simulink library "relay_ANSI_functions_lib"  (Simulink 8.1)
settings: Solver=ode45  StartTime=0.0  StopTime=10.0  RelTol=1e-3
values from neighbouring files (symbols this model uses):
  Ts = 100E-6    (= 0.0001)    [UnitTest_relay_model_init.m]    (also in relay_settings_init.m)
undefined symbols (not defined in the file or in its folder): IOC, TOC, VRMSLL
libraries: simulink x4
settings Model: Creator=RE25624  LastModifiedBy=re25624

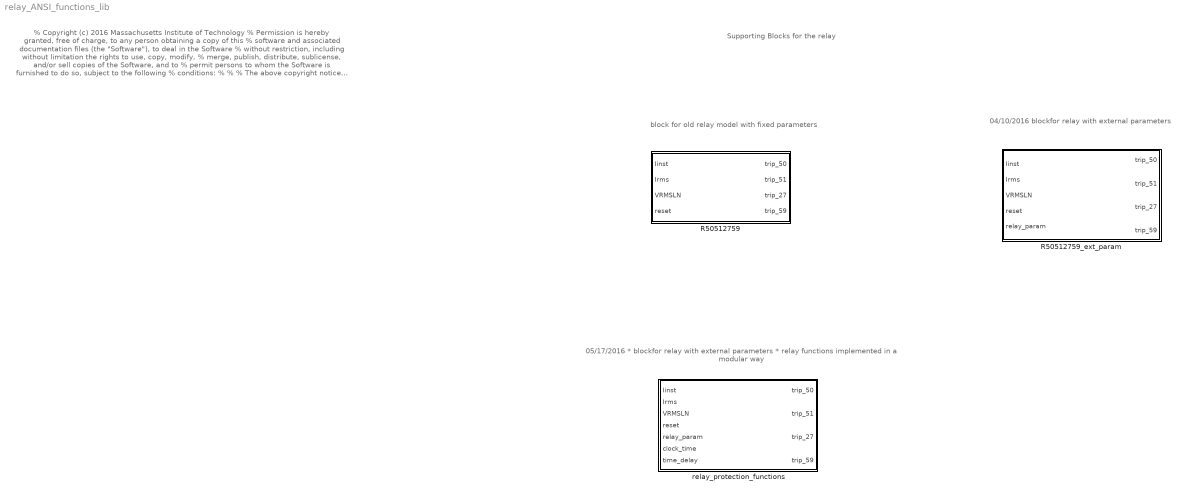
== system relay_ANSI_functions_lib ==
  note: 04/10/2016
      | blockfor relay with external parameters
  note: Supporting Blocks for the relay
  note: block for old relay model with fixed parameters
  note: 05/17/2016
      | * blockfor relay with external parameters
      | * relay functions implemented in a modular way
  note: % Copyright (c) 2016 Massachusetts Institute of Technology
      | % Permission is hereby granted, free of charge, to any person obtaining a copy of this
      | % software and associated documentation files (the "Software"), to deal in the Software
      | % without restriction, including without limitation the rights to use, copy, modify,
      | % merge, publish, distribute, sublicense, and/or sell copies of the Software, and to
      | % permit persons to whom the Software is furnished to do so, subject to the following
      | % conditions:
      | %
      | %
      | % The above copyright notice and this permission notice shall be included in
      | % all copies or substantial portions of the Software.
      | %
      | % THE SOFTWARE IS PROVIDED "AS IS", WITHOUT WARRANTY OF ANY KIND, EXPRESS OR IMPLIED,
      | % INCLUDING BUT NOT LIMITED TO THE WARRANTIES OF MERCHANTABILITY, FITNESS FOR A
      | % PARTICULAR PURPOSE AND NONINFRINGEMENT. IN NO EVENT SHALL THE AUTHORS OR COPYRIGHT
      | % HOLDERS BE LIABLE FOR ANY CLAIM, DAMAGES OR OTHER LIABILITY, WHETHER IN AN ACTION
      | % OF CONTRACT, TORT OR OTHERWISE, ARISING FROM, OUT OF OR IN CONNECTION WITH THE
      | % SOFTWARE OR THE USE OR OTHER DEALINGS IN THE SOFTWARE.
      | %
      | %
      | %%
  R50512759 : Subsystem  mask(Relays 50-51-27-59){VRMSLL=VRMSLL, IOC=IOC, TOC=TOC, Ts=Ts}
      mask prompts: VRMSLL "Nominal Voltage [VRMSLL]"; IOC "IOC Setting [A]"; TOC "TOC Setting [A]"; Ts "Sampling Time [Sec]"
      mask help:
      | This block simulates the behavior of the following relay functions:
      | 1) Instantaneous overcurrent (50)
      | 2) AC inverse time overcurrent (51)
      | 3) Undervoltage (27)
      | 4) Overvoltage (59)
      | It is not suitable for instantaneous earth current relaying.
      | The model neglects the influence CTs since only the logics of the relay are required or the current effort.
  R50512759_ext_param : Subsystem  mask(Relays 50-51-27-59){Ts=Ts}
      mask prompts: Ts "Sampling Time [Sec]"
      mask help:
      | This block simulates the behavior of the following relay functions:
      | 1) Instantaneous overcurrent (50)
      | 2) AC inverse time overcurrent (51)
      | 3) Undervoltage (27)
      | 4) Overvoltage (59)
      | It is not suitable for instantaneous earth current relaying.
      | The model neglects the influence CTs since only the logics of the relay are required or the current effort.
      |
      | The input bus with the relay parameters should be ordered as follows:
      | 1) VRMSLL
      | 2) IOC
      | 3) TOC
      | 4) dV_threshold
      | 5) angle_threshold
      | 6) dF_threshold
  relay_protection_functions : Subsystem  mask(Relays 50-51-27-59){Ts=Ts}
      mask prompts: Ts "Sampling Time [Sec]"
      mask help:
      | This block simulates the behavior of the following relay functions:
      | 1) Instantaneous overcurrent (50)
      | 2) AC inverse time overcurrent (51)
      | 3) Undervoltage (27)
      | 4) Overvoltage (59)
      | It is not suitable for instantaneous earth current relaying.
      | The model neglects the influence CTs since only the logics of the relay are required or the current effort.
      |
      | The input bus with the relay parameters should be ordered as follows:
      | 1) VRMSLL
      | 2) IOC
      | 3) TOC
      | 4) dV_threshold
      | 5) angle_threshold
      | 6) dF_threshold

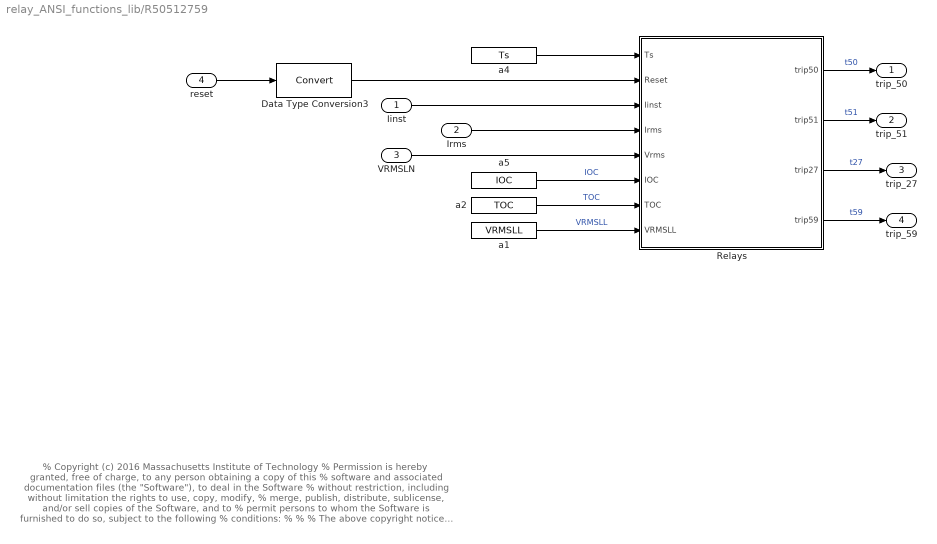
== system relay_ANSI_functions_lib/R50512759 ==
  note: % Copyright (c) 2016 Massachusetts Institute of Technology
      | % Permission is hereby granted, free of charge, to any person obtaining a copy of this
      | % software and associated documentation files (the "Software"), to deal in the Software
      | % without restriction, including without limitation the rights to use, copy, modify,
      | % merge, publish, distribute, sublicense, and/or sell copies of the Software, and to
      | % permit persons to whom the Software is furnished to do so, subject to the following
      | % conditions:
      | %
      | %
      | % The above copyright notice and this permission notice shall be included in
      | % all copies or substantial portions of the Software.
      | %
      | % THE SOFTWARE IS PROVIDED "AS IS", WITHOUT WARRANTY OF ANY KIND, EXPRESS OR IMPLIED,
      | % INCLUDING BUT NOT LIMITED TO THE WARRANTIES OF MERCHANTABILITY, FITNESS FOR A
      | % PARTICULAR PURPOSE AND NONINFRINGEMENT. IN NO EVENT SHALL THE AUTHORS OR COPYRIGHT
      | % HOLDERS BE LIABLE FOR ANY CLAIM, DAMAGES OR OTHER LIABILITY, WHETHER IN AN ACTION
      | % OF CONTRACT, TORT OR OTHERWISE, ARISING FROM, OUT OF OR IN CONNECTION WITH THE
      | % SOFTWARE OR THE USE OR OTHER DEALINGS IN THE SOFTWARE.
      | %
      | %
      | %%
  Iinst : Inport
  Irms : Inport  Port=2
  VRMSLN : Inport  Port=3
  reset : Inport  Port=4
  Data Type Conversion3 : DataTypeConversion
  Relays : MATLAB Function  TreatAsAtomicUnit=on
  a1 : Constant  Value=VRMSLL
  a2 : Constant  Value=TOC
  a4 : Constant  Value=Ts
  a5 : Constant  Value=IOC
  trip_50 : Outport
  trip_51 : Outport  Port=2
  trip_27 : Outport  Port=3
  trip_59 : Outport  Port=4
  wires:
  Data Type Conversion3/1 -> Relays/2(Reset)
  Relays/2(trip51) -> trip_51/1  "t51"
  Relays/1(trip50) -> trip_50/1  "t50"
  Relays/4(trip59) -> trip_59/1  "t59"
  Relays/3(trip27) -> trip_27/1  "t27"
  a4/1 -> Relays/1(Ts)
  a1/1 -> Relays/8(VRMSLL)  "VRMSLL"
  VRMSLN/1 -> Relays/5(Vrms)
  Irms/1 -> Relays/4(Irms)
  a2/1 -> Relays/7(TOC)  "TOC"
  Iinst/1 -> Relays/3(Iinst)
  a5/1 -> Relays/6(IOC)  "IOC"
  reset/1 -> Data Type Conversion3/1

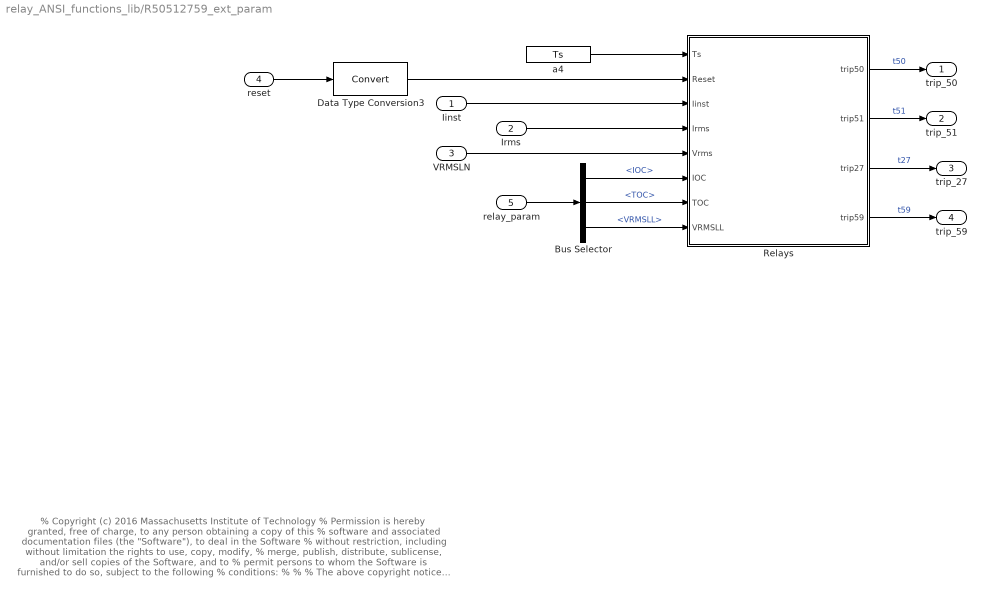
== system relay_ANSI_functions_lib/R50512759_ext_param ==
  note: % Copyright (c) 2016 Massachusetts Institute of Technology
      | % Permission is hereby granted, free of charge, to any person obtaining a copy of this
      | % software and associated documentation files (the "Software"), to deal in the Software
      | % without restriction, including without limitation the rights to use, copy, modify,
      | % merge, publish, distribute, sublicense, and/or sell copies of the Software, and to
      | % permit persons to whom the Software is furnished to do so, subject to the following
      | % conditions:
      | %
      | %
      | % The above copyright notice and this permission notice shall be included in
      | % all copies or substantial portions of the Software.
      | %
      | % THE SOFTWARE IS PROVIDED "AS IS", WITHOUT WARRANTY OF ANY KIND, EXPRESS OR IMPLIED,
      | % INCLUDING BUT NOT LIMITED TO THE WARRANTIES OF MERCHANTABILITY, FITNESS FOR A
      | % PARTICULAR PURPOSE AND NONINFRINGEMENT. IN NO EVENT SHALL THE AUTHORS OR COPYRIGHT
      | % HOLDERS BE LIABLE FOR ANY CLAIM, DAMAGES OR OTHER LIABILITY, WHETHER IN AN ACTION
      | % OF CONTRACT, TORT OR OTHERWISE, ARISING FROM, OUT OF OR IN CONNECTION WITH THE
      | % SOFTWARE OR THE USE OR OTHER DEALINGS IN THE SOFTWARE.
      | %
      | %
      | %%
  Iinst : Inport
  Irms : Inport  Port=2
  VRMSLN : Inport  Port=3
  reset : Inport  Port=4
  relay_param : Inport  Port=5
  Bus Selector : BusSelector  OutputSignals=IOC,TOC,VRMSLL
  Data Type Conversion3 : DataTypeConversion
  Relays : MATLAB Function  TreatAsAtomicUnit=on
  a4 : Constant  Value=Ts
  trip_50 : Outport
  trip_51 : Outport  Port=2
  trip_27 : Outport  Port=3
  trip_59 : Outport  Port=4
  wires:
  relay_param/1 -> Bus Selector/1
  Data Type Conversion3/1 -> Relays/2(Reset)
  Relays/2(trip51) -> trip_51/1  "t51"
  Relays/1(trip50) -> trip_50/1  "t50"
  Relays/4(trip59) -> trip_59/1  "t59"
  Relays/3(trip27) -> trip_27/1  "t27"
  a4/1 -> Relays/1(Ts)
  Bus Selector/3 -> Relays/8(VRMSLL)  "<VRMSLL>"
  VRMSLN/1 -> Relays/5(Vrms)
  Irms/1 -> Relays/4(Irms)
  Bus Selector/2 -> Relays/7(TOC)  "<TOC>"
  Iinst/1 -> Relays/3(Iinst)
  Bus Selector/1 -> Relays/6(IOC)  "<IOC>"
  reset/1 -> Data Type Conversion3/1

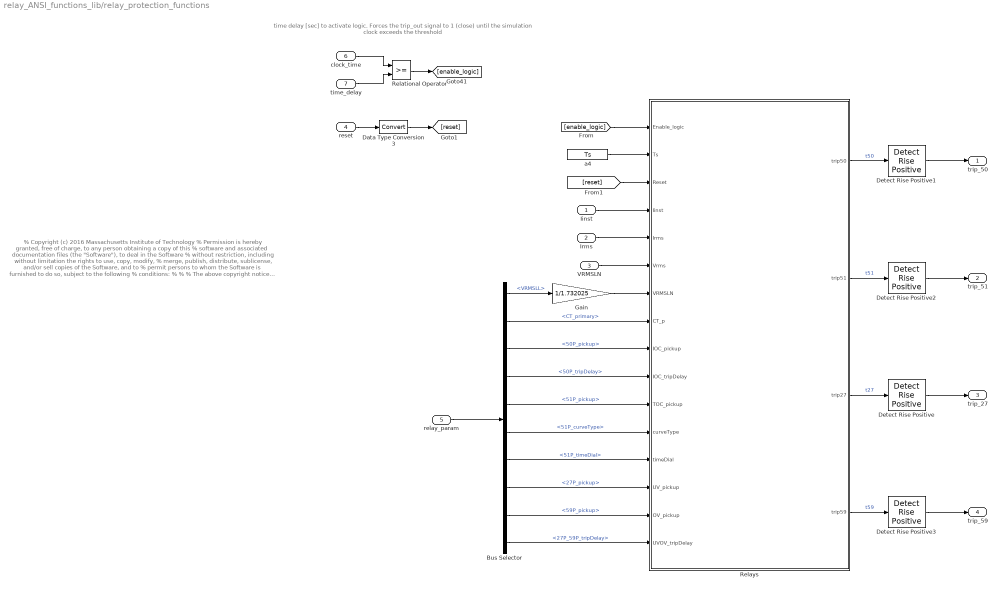
== system relay_ANSI_functions_lib/relay_protection_functions ==
  note: time delay [sec] to activate logic. Forces the trip_out signal
      | to 1 (close) until the simulation clock exceeds the threshold
  note: % Copyright (c) 2016 Massachusetts Institute of Technology
      | % Permission is hereby granted, free of charge, to any person obtaining a copy of this
      | % software and associated documentation files (the "Software"), to deal in the Software
      | % without restriction, including without limitation the rights to use, copy, modify,
      | % merge, publish, distribute, sublicense, and/or sell copies of the Software, and to
      | % permit persons to whom the Software is furnished to do so, subject to the following
      | % conditions:
      | %
      | %
      | % The above copyright notice and this permission notice shall be included in
      | % all copies or substantial portions of the Software.
      | %
      | % THE SOFTWARE IS PROVIDED "AS IS", WITHOUT WARRANTY OF ANY KIND, EXPRESS OR IMPLIED,
      | % INCLUDING BUT NOT LIMITED TO THE WARRANTIES OF MERCHANTABILITY, FITNESS FOR A
      | % PARTICULAR PURPOSE AND NONINFRINGEMENT. IN NO EVENT SHALL THE AUTHORS OR COPYRIGHT
      | % HOLDERS BE LIABLE FOR ANY CLAIM, DAMAGES OR OTHER LIABILITY, WHETHER IN AN ACTION
      | % OF CONTRACT, TORT OR OTHERWISE, ARISING FROM, OUT OF OR IN CONNECTION WITH THE
      | % SOFTWARE OR THE USE OR OTHER DEALINGS IN THE SOFTWARE.
      | %
      | %
      | %%
  Iinst : Inport
  Irms : Inport  Port=2
  VRMSLN : Inport  Port=3
  reset : Inport  Port=4
  relay_param : Inport  Port=5
  clock_time : Inport  Port=6
  time_delay : Inport  Port=7
  Bus Selector : BusSelector  OutputSignals=VRMSLL,CT_primary,50P_pickup,50P_tripDelay,51P_pickup,51P_curveType,51P_timeDial,27P_pickup,59P_pickup,27P_59P_tripDelay
  Data Type Conversion3 : DataTypeConversion
  Detect Rise Positive{,1..3} (4 alike) : simulink/Logic and Bit Operations/Detect Rise Positive  vinit=0  InputProcessing=Inherited  OutDataTypeStr=boolean
  Gain : Gain  Gain=1/1.732025
  Relational Operator : RelationalOperator  OutDataTypeStr=boolean
  Relays : MATLAB Function  TreatAsAtomicUnit=on
  a4 : Constant  Value=Ts
  trip_50 : Outport
  trip_51 : Outport  Port=2
  trip_27 : Outport  Port=3
  trip_59 : Outport  Port=4
  wires:
  Detect Rise Positive3/1 -> trip_59/1
  Detect Rise Positive/1 -> trip_27/1
  Detect Rise Positive2/1 -> trip_51/1
  Detect Rise Positive1/1 -> trip_50/1
  Relays/4(trip59) -> Detect Rise Positive3/1  "t59"
  Relays/2(trip51) -> Detect Rise Positive2/1  "t51"
  Relays/1(trip50) -> Detect Rise Positive1/1  "t50"
  Relays/3(trip27) -> Detect Rise Positive/1  "t27"
  [reset] -> Relays/3(Reset)
  Data Type Conversion3/1 -> [reset]
  Gain/1 -> Relays/7(VRMSLN)
  Bus Selector/8 -> Relays/14(UV_pickup)  "<27P_pickup>"
  Bus Selector/9 -> Relays/15(OV_pickup)  "<59P_pickup>"
  Bus Selector/10 -> Relays/16(UVOV_tripDelay)  "<27P_59P_tripDelay>"
  Iinst/1 -> Relays/4(Iinst)
  Irms/1 -> Relays/5(Irms)
  Bus Selector/7 -> Relays/13(timeDial)  "<51P_timeDial>"
  Bus Selector/6 -> Relays/12(curveType)  "<51P_curveType>"
  Bus Selector/5 -> Relays/11(TOC_pickup)  "<51P_pickup>"
  Bus Selector/4 -> Relays/10(IOC_tripDelay)  "<50P_tripDelay>"
  Bus Selector/3 -> Relays/9(IOC_pickup)  "<50P_pickup>"
  Bus Selector/2 -> Relays/8(CT_p)  "<CT_primary>"
  Bus Selector/1 -> Gain/1  "<VRMSLL>"
  reset/1 -> Data Type Conversion3/1
  VRMSLN/1 -> Relays/6(Vrms)
  a4/1 -> Relays/2(Ts)
  relay_param/1 -> Bus Selector/1
  clock_time/1 -> Relational Operator/1
  time_delay/1 -> Relational Operator/2
  Relational Operator/1 -> [enable_logic]
  [enable_logic] -> Relays/1(Enable_logic)

== matlab function relay_protection_functions/Relays ==
  data: Enable_logic input double; Ts input double; Reset input double; Iinst input double; Irms input double; Vrms input double; VRMSLN input double; CT_p input double; IOC_pickup input double; IOC_tripDelay input double; TOC_pickup input double; curveType input double; timeDial input double; UV_pickup input double; OV_pickup input double; UVOV_tripDelay input double; trip50 output double; trip51 output double; trip27 output double; trip59 output double
% Copyright (c) 2016 Massachusetts Institute of Technology
% Permission is hereby granted, free of charge, to any person obtaining a copy of this
% software and associated documentation files (the "Software"), to deal in the Software
% without restriction, including without limitation the rights to use, copy, modify,
% merge, publish, distribute, sublicense, and/or sell copies of the Software, and to
% permit persons to whom the Software is furnished to do so, subject to the following
% conditions:
%
%
% The above copyright notice and this permission notice shall be included in
% all copies or substantial portions of the Software.
%
% THE SOFTWARE IS PROVIDED "AS IS", WITHOUT WARRANTY OF ANY KIND, EXPRESS OR IMPLIED,
% INCLUDING BUT NOT LIMITED TO THE WARRANTIES OF MERCHANTABILITY, FITNESS FOR A
% PARTICULAR PURPOSE AND NONINFRINGEMENT. IN NO EVENT SHALL THE AUTHORS OR COPYRIGHT
% HOLDERS BE LIABLE FOR ANY CLAIM, DAMAGES OR OTHER LIABILITY, WHETHER IN AN ACTION
% OF CONTRACT, TORT OR OTHERWISE, ARISING FROM, OUT OF OR IN CONNECTION WITH THE
% SOFTWARE OR THE USE OR OTHER DEALINGS IN THE SOFTWARE.
%
%
%%

function [trip50, trip51, trip27, trip59] = relay_elements(Enable_logic, Ts, Reset, Iinst, Irms, Vrms, VRMSLN,...
    CT_p, IOC_pickup, IOC_tripDelay, TOC_pickup, curveType, timeDial, UV_pickup, OV_pickup, UVOV_tripDelay)
%#codegen

% initialize or reset the trip signals
persistent R50 R51 R27 R59
if isempty(R51) || Reset
    R50=false;
    R51=false;
    R59=false;
    R27=false;
end

% applying turns CT ratio - assuming protection type CT
Iinst = Iinst * (5/CT_p);
Irms = Irms * (5/CT_p);

% old- latch for true signals
% old- if ~(R50==true || R51==true) && Enable_logic==1
if Enable_logic==1
    % calling external function expressing relay protection elements
    T50 = relay_ANSI_50P_script(Ts, Iinst , IOC_pickup, IOC_tripDelay);
    T51 = relay_ANSI_51P_script(Ts, Irms, TOC_pickup, curveType, timeDial);
    T27 = relay_ANSI_27P_script(Ts, Vrms, VRMSLN, UV_pickup, UVOV_tripDelay);
    T59 = relay_ANSI_59P_script(Ts, Vrms, VRMSLN, OV_pickup, UVOV_tripDelay);
    
    R50 = T50;
    R51 = T51;
    R27 = T27;
    R59 = T59;
end

% external latch
trip50 = R50; % old- latched
trip51 = R51; % old- latched
trip27 = R27; % old- not latched
trip59 = R59; % old- not latched

== matlab function R50512759/Relays ==
  data: Ts input double; trip50 output double; Reset input double; Iinst input double; Irms input double; Vrms input double; IOC input double; trip51 output double; trip27 output double; TOC input double; VRMSLL input double; trip59 output double
% Copyright (c) 2016 Massachusetts Institute of Technology
% Permission is hereby granted, free of charge, to any person obtaining a copy of this 
% software and associated documentation files (the "Software"), to deal in the Software
% without restriction, including without limitation the rights to use, copy, modify, 
% merge, publish, distribute, sublicense, and/or sell copies of the Software, and to 
% permit persons to whom the Software is furnished to do so, subject to the following 
% conditions:
% 
% 
% The above copyright notice and this permission notice shall be included in 
% all copies or substantial portions of the Software.
% 
% THE SOFTWARE IS PROVIDED "AS IS", WITHOUT WARRANTY OF ANY KIND, EXPRESS OR IMPLIED, 
% INCLUDING BUT NOT LIMITED TO THE WARRANTIES OF MERCHANTABILITY, FITNESS FOR A 
% PARTICULAR PURPOSE AND NONINFRINGEMENT. IN NO EVENT SHALL THE AUTHORS OR COPYRIGHT 
% HOLDERS BE LIABLE FOR ANY CLAIM, DAMAGES OR OTHER LIABILITY, WHETHER IN AN ACTION 
% OF CONTRACT, TORT OR OTHERWISE, ARISING FROM, OUT OF OR IN CONNECTION WITH THE 
% SOFTWARE OR THE USE OR OTHER DEALINGS IN THE SOFTWARE.
%
%
%%


function [trip50, trip51, trip27, trip59] = relays_50512759(Ts, Reset, Iinst, Irms, Vrms, IOC, TOC, VRMSLL)
%#codegen

% initialize or reset the trip signals
persistent R50 R51 R27 R59
if isempty(R51) || Reset
    R50=false;
    R51=false;
    R59=false;
    R27=false;
end

% latch for true signals
if ~(R50==true || R51==true)
    % calling external function
    r = relay_ANSI_50512759_script(Ts, Iinst, Irms, Vrms, IOC, TOC, VRMSLL);
    R50 = r.trip50;
    R51 = r.trip51;
    R27 = r.trip27;
    R59 = r.trip59;
end

trip50 = R50; % latched
trip51 = R51; % latched
trip27 = R27; % not latched
trip59 = R59; % not latched

== matlab function R50512759_ext_param/Relays ==
  data: Ts input double; trip50 output double; Reset input double; Iinst input double; Irms input double; Vrms input double; IOC input double; trip51 output double; trip27 output double; TOC input double; VRMSLL input double; trip59 output double
% Copyright (c) 2016 Massachusetts Institute of Technology
% Permission is hereby granted, free of charge, to any person obtaining a copy of this 
% software and associated documentation files (the "Software"), to deal in the Software
% without restriction, including without limitation the rights to use, copy, modify, 
% merge, publish, distribute, sublicense, and/or sell copies of the Software, and to 
% permit persons to whom the Software is furnished to do so, subject to the following 
% conditions:
% 
% 
% The above copyright notice and this permission notice shall be included in 
% all copies or substantial portions of the Software.
% 
% THE SOFTWARE IS PROVIDED "AS IS", WITHOUT WARRANTY OF ANY KIND, EXPRESS OR IMPLIED, 
% INCLUDING BUT NOT LIMITED TO THE WARRANTIES OF MERCHANTABILITY, FITNESS FOR A 
% PARTICULAR PURPOSE AND NONINFRINGEMENT. IN NO EVENT SHALL THE AUTHORS OR COPYRIGHT 
% HOLDERS BE LIABLE FOR ANY CLAIM, DAMAGES OR OTHER LIABILITY, WHETHER IN AN ACTION 
% OF CONTRACT, TORT OR OTHERWISE, ARISING FROM, OUT OF OR IN CONNECTION WITH THE 
% SOFTWARE OR THE USE OR OTHER DEALINGS IN THE SOFTWARE.
%
%
%%

function [trip50, trip51, trip27, trip59] = relays_50512759(Ts, Reset, Iinst, Irms, Vrms, IOC, TOC, VRMSLL)
%#codegen

% initialize or reset the trip signals
persistent R50 R51 R27 R59
if isempty(R51) || Reset
    R50=false;
    R51=false;
    R59=false;
    R27=false;
end

% latch for true signals
if ~(R50==true || R51==true)
    % calling external function
    r = relay_ANSI_50512759_script(Ts, Iinst, Irms, Vrms, IOC, TOC, VRMSLL);
    R50 = r.trip50;
    R51 = r.trip51;
    R27 = r.trip27;
    R59 = r.trip59;
end

trip50 = R50; % latched
trip51 = R51; % latched
trip27 = R27; % not latched
trip59 = R59; % not latched
